simulink model "Buck_DCM_s"  (R2020a)
settings: Solver=FixedStepAuto  StartTime=0.0  StopTime=1  FixedStep=T  RelTol=1e-3
undefined symbols (not defined in the file): C, Idm, Iumax, J, Ki_I, Ki_IL, Ki_W, Kp_I, Kp_IL, Kp_Uc, Kp_W, Kphi, L, Lu, rL, Ru, Ubat
libraries: fl_lib x7, simulink x6, nesl_utility x3, powerlib_meascontrol x2
settings Model: SILPILModeSetting=veronly  ExtModeTrigDuration=2  Creator=Nguyễn Thanh Tùng  LastModifiedBy=Nguyen Tung
settings OptimizationCC: DefaultParameterBehavior=Inlined  EnhancedBackFolding=on  PassReuseOutputArgsAs=Individual arguments  ZeroExternalMemoryAtStartup=off  ZeroInternalMemoryAtStartup=off  MaxStackSize=64  OptimizeBlockOrder=speed  DifferentSizesBufferReuse=on  OptimizationCustomize=off  EfficientTunableParamExpr=on
settings DebuggingCC: ParameterTunabilityLossMsg=error
settings SFSimCC: MATLABDynamicMemAlloc=off  CustomCodeUndefinedFunction=UseInterfaceOnly
settings RTWCC: SystemTargetFile=ert.tlc  TemplateMakefile=ert_default_tmf  Toolchain=Arduino ARM  BuildConfiguration=Faster Runs
settings CodeAppCC: ForceParamTrailComments=on  IgnoreCustomStorageClasses=off  OperatorAnnotations=on  SimulinkDataObjDesc=on  SFDataObjDesc=on  InsertBlockDesc=on
settings ERTTargetCC: SupportContinuousTime=on  ExtModeStaticAllocSize=24576  ERTCustomFileTemplate=example_file_process.tlc

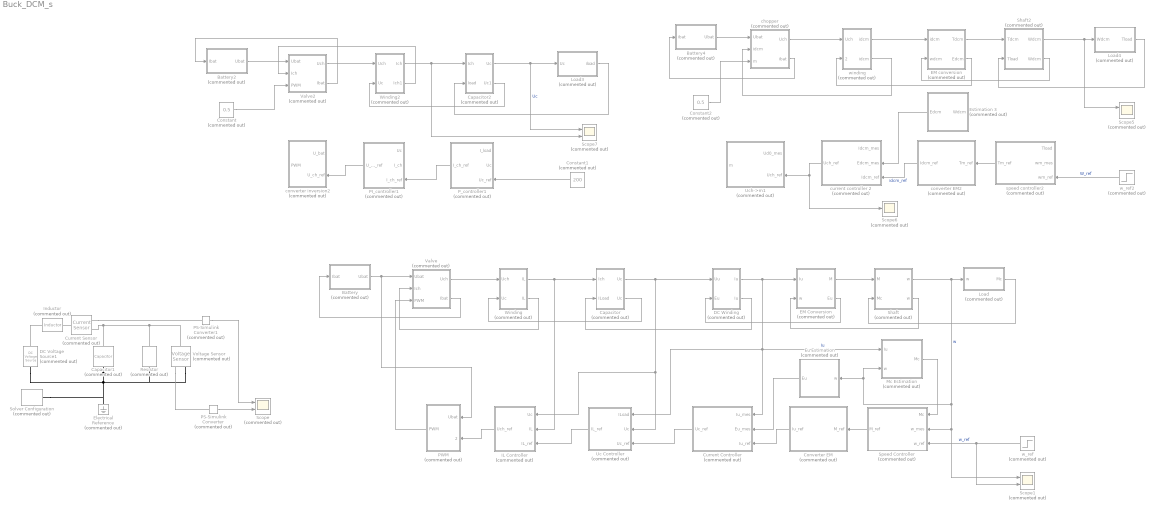
== system Buck_DCM_s ==
  Battery : Subsystem  Commented=on  AncestorBlock=simulink/REM/SE
      mask Display:
      | plot(0,0,100,100, 1.2*[50,57.68,60.77,63.08,64.97,66.58,68,69.26,70.4, 	71.42,72.36,78.28,80,78.28,72.36,71.42,70.4, 	69.26,68,66.58,64.97,63.08,60.77,57.68,50,42.32, 	39.23,36.92,35.03,33.42,32,30.74,29.6,28.58, 	27.64,21.72,20,21.72,27.64,28.58,29.6,30.74,32, 	33.42,35.03,36.92,39.23,42.32,50]-10, 1.2*[20,21,22,23,24,25,26,27,28,29,30,40,50,60,70,71,72, 	73,74,75,76,77,78,79,80,79,78,77,76,75,74,73,72, 	71,70,60,50,40,30,29,28,27,26,25,24,23,22,21,20]-10)
      | disp('ES')
  Battery2 : Subsystem  Commented=on  AncestorBlock=simulink/REM/SE
      mask Display:
      | plot(0,0,100,100, 1.2*[50,57.68,60.77,63.08,64.97,66.58,68,69.26,70.4, 	71.42,72.36,78.28,80,78.28,72.36,71.42,70.4, 	69.26,68,66.58,64.97,63.08,60.77,57.68,50,42.32, 	39.23,36.92,35.03,33.42,32,30.74,29.6,28.58, 	27.64,21.72,20,21.72,27.64,28.58,29.6,30.74,32, 	33.42,35.03,36.92,39.23,42.32,50]-10, 1.2*[20,21,22,23,24,25,26,27,28,29,30,40,50,60,70,71,72, 	73,74,75,76,77,78,79,80,79,78,77,76,75,74,73,72, 	71,70,60,50,40,30,29,28,27,26,25,24,23,22,21,20]-10)
      | disp('ES')
  Battery4 : Subsystem  Commented=on  AncestorBlock=simulink/REM/SE
      mask Display:
      | plot(0,0,100,100, 1.2*[50,57.68,60.77,63.08,64.97,66.58,68,69.26,70.4, 	71.42,72.36,78.28,80,78.28,72.36,71.42,70.4, 	69.26,68,66.58,64.97,63.08,60.77,57.68,50,42.32, 	39.23,36.92,35.03,33.42,32,30.74,29.6,28.58, 	27.64,21.72,20,21.72,27.64,28.58,29.6,30.74,32, 	33.42,35.03,36.92,39.23,42.32,50]-10, 1.2*[20,21,22,23,24,25,26,27,28,29,30,40,50,60,70,71,72, 	73,74,75,76,77,78,79,80,79,78,77,76,75,74,73,72, 	71,70,60,50,40,30,29,28,27,26,25,24,23,22,21,20]-10)
      | disp('ES')
  Capacitor : Subsystem  Commented=on  AncestorBlock=simulink/REM/EA  mask(CM){}
      mask Display: plot(0,0,100,100,[10,10,90,90,10],[90,10,10,90,90], [10,90],[10,90])
  Capacitor1 : fl_lib/Electrical/Electrical Elements/Capacitor  Commented=on  c=C F  r=0 Ohm  g=0 1/Ohm  i_specify=off  i_priority=None  i=0 A  i_nominal_specify=off  i_nominal_unit=A  i_nominal_value=1  v_specify=off  v_priority=None  v=0 V  v_nominal_specify=off  v_nominal_unit=V  v_nominal_value=1  vc_specify=off  vc_priority=High  vc=0 V  vc_nominal_specify=off  vc_nominal_unit=V  vc_nominal_value=1
  Capacitor2 : Subsystem  Commented=on  AncestorBlock=simulink/REM/EA  mask(CM){}
      mask Display: plot(0,0,100,100,[10,10,90,90,10],[90,10,10,90,90], [10,90],[10,90])
  Constant : Constant  Commented=on  Value=0.5
  Constant1 : Constant  Commented=on  Value=200
  Constant2 : Constant  Commented=on  Value=0.5
  Converter EM : Subsystem  Commented=on  AncestorBlock=simulink/SMC/Inversion EC avec mesure
      mask Display: plot(0,0,100,100,[10,30,90,70,10],[90,10,10,90,90])
  Current Controller : Subsystem  Commented=on  AncestorBlock=simulink/SMC/Asservissement Correcteur IP
      mask Display: plot(0,0,100,100, [10,30,90,70,10,90],[90,10,10,90,90,10])
  Current Sensor : fl_lib/Electrical/Electrical Sensors/Current Sensor  Commented=on
  DC Voltage Source1 : fl_lib/Electrical/Electrical Sources/DC Voltage Source  Commented=on  v0=100 V
  DC Winding : Subsystem  Commented=on  AncestorBlock=simulink/REM/EA  mask(CM){}
      mask Display: plot(0,0,100,100,[10,10,90,90,10],[90,10,10,90,90], [10,90],[10,90])
  EM Conversion : Subsystem  Commented=on  AncestorBlock=simulink/REM/EC EM
      mask Display: plot(0,0,100,100, 1.4*[50,57.68,60.77,63.08,64.97,66.58,68,69.26,70.4, 	71.42,72.36,78.28,80,78.28,72.36,71.42,70.4, 	69.26,68,66.58,64.97,63.08,60.77,57.68,50,42.32, 	39.23,36.92,35.03,33.42,32,30.74,29.6,28.58, 	27.64,21.72,20,21.72,27.64,28.58,29.6,30.74,32, 	33.42,35.03,36.92,39.23,42.32,50]-20, 1.4*[20,21,22,23,24,25,26,27,28,29,30,40,50,60,70,71,72, 	73,74,75,76,77,78,79,80,79,78,77,76,75,74,73,72, 	71,70,60,50,40,30,29,28,27,26,25,24,23,22,21,20]-20)
  EM conversion : Subsystem  Commented=on  AncestorBlock=simulink/REM/EC EM
      mask Display: plot(0,0,100,100, 1.4*[50,57.68,60.77,63.08,64.97,66.58,68,69.26,70.4, 	71.42,72.36,78.28,80,78.28,72.36,71.42,70.4, 	69.26,68,66.58,64.97,63.08,60.77,57.68,50,42.32, 	39.23,36.92,35.03,33.42,32,30.74,29.6,28.58, 	27.64,21.72,20,21.72,27.64,28.58,29.6,30.74,32, 	33.42,35.03,36.92,39.23,42.32,50]-20, 1.4*[20,21,22,23,24,25,26,27,28,29,30,40,50,60,70,71,72, 	73,74,75,76,77,78,79,80,79,78,77,76,75,74,73,72, 	71,70,60,50,40,30,29,28,27,26,25,24,23,22,21,20]-20)
  Electrical Reference : fl_lib/Electrical/Electrical Elements/Electrical Reference  Commented=on
  Estimation 3 : Subsystem  Commented=on  AncestorBlock=simulink/REM/EC EM
      mask Display: plot(0,0,100,100, 1.4*[50,57.68,60.77,63.08,64.97,66.58,68,69.26,70.4, 	71.42,72.36,78.28,80,78.28,72.36,71.42,70.4, 	69.26,68,66.58,64.97,63.08,60.77,57.68,50,42.32, 	39.23,36.92,35.03,33.42,32,30.74,29.6,28.58, 	27.64,21.72,20,21.72,27.64,28.58,29.6,30.74,32, 	33.42,35.03,36.92,39.23,42.32,50]-20, 1.4*[20,21,22,23,24,25,26,27,28,29,30,40,50,60,70,71,72, 	73,74,75,76,77,78,79,80,79,78,77,76,75,74,73,72, 	71,70,60,50,40,30,29,28,27,26,25,24,23,22,21,20]-20)
  Eu Estimation : Subsystem  Commented=on  AncestorBlock=simulink/REM/EC EM
      mask Display: plot(0,0,100,100, 1.4*[50,57.68,60.77,63.08,64.97,66.58,68,69.26,70.4, 	71.42,72.36,78.28,80,78.28,72.36,71.42,70.4, 	69.26,68,66.58,64.97,63.08,60.77,57.68,50,42.32, 	39.23,36.92,35.03,33.42,32,30.74,29.6,28.58, 	27.64,21.72,20,21.72,27.64,28.58,29.6,30.74,32, 	33.42,35.03,36.92,39.23,42.32,50]-20, 1.4*[20,21,22,23,24,25,26,27,28,29,30,40,50,60,70,71,72, 	73,74,75,76,77,78,79,80,79,78,77,76,75,74,73,72, 	71,70,60,50,40,30,29,28,27,26,25,24,23,22,21,20]-20)
  IL Controller : Subsystem  Commented=on  AncestorBlock=simulink/SMC/Asservissement Correcteur IP
      mask Display: plot(0,0,100,100, [10,30,90,70,10,90],[90,10,10,90,90,10])
  Inductor : fl_lib/Electrical/Electrical Elements/Inductor  Commented=on  l=L H  r=rL Ohm  g=0 1/Ohm  i_specify=off  i_priority=None  i=0 A  i_nominal_specify=off  i_nominal_unit=A  i_nominal_value=1  v_specify=off  v_priority=None  v=0 V  v_nominal_specify=off  v_nominal_unit=V  v_nominal_value=1  i_L_specify=off  i_L_priority=High  i_L=0 A  i_L_nominal_specify=off  i_L_nominal_unit=A  i_L_nominal_value=1
  Load : Subsystem  Commented=on  AncestorBlock=simulink/REM/SE
      mask Display:
      | plot(0,0,100,100, 1.2*[50,57.68,60.77,63.08,64.97,66.58,68,69.26,70.4, 	71.42,72.36,78.28,80,78.28,72.36,71.42,70.4, 	69.26,68,66.58,64.97,63.08,60.77,57.68,50,42.32, 	39.23,36.92,35.03,33.42,32,30.74,29.6,28.58, 	27.64,21.72,20,21.72,27.64,28.58,29.6,30.74,32, 	33.42,35.03,36.92,39.23,42.32,50]-10, 1.2*[20,21,22,23,24,25,26,27,28,29,30,40,50,60,70,71,72, 	73,74,75,76,77,78,79,80,79,78,77,76,75,74,73,72, 	71,70,60,50,40,30,29,28,27,26,25,24,23,22,21,20]-10)
      | disp('MS')
  Load3 : Subsystem  Commented=on  AncestorBlock=simulink/REM/SE
      mask Display:
      | plot(0,0,100,100, 1.2*[50,57.68,60.77,63.08,64.97,66.58,68,69.26,70.4, 	71.42,72.36,78.28,80,78.28,72.36,71.42,70.4, 	69.26,68,66.58,64.97,63.08,60.77,57.68,50,42.32, 	39.23,36.92,35.03,33.42,32,30.74,29.6,28.58, 	27.64,21.72,20,21.72,27.64,28.58,29.6,30.74,32, 	33.42,35.03,36.92,39.23,42.32,50]-10, 1.2*[20,21,22,23,24,25,26,27,28,29,30,40,50,60,70,71,72, 	73,74,75,76,77,78,79,80,79,78,77,76,75,74,73,72, 	71,70,60,50,40,30,29,28,27,26,25,24,23,22,21,20]-10)
      | disp('ES')
  Load4 : Subsystem  Commented=on  AncestorBlock=simulink/REM/SE
      mask Display:
      | plot(0,0,100,100, 1.2*[50,57.68,60.77,63.08,64.97,66.58,68,69.26,70.4, 	71.42,72.36,78.28,80,78.28,72.36,71.42,70.4, 	69.26,68,66.58,64.97,63.08,60.77,57.68,50,42.32, 	39.23,36.92,35.03,33.42,32,30.74,29.6,28.58, 	27.64,21.72,20,21.72,27.64,28.58,29.6,30.74,32, 	33.42,35.03,36.92,39.23,42.32,50]-10, 1.2*[20,21,22,23,24,25,26,27,28,29,30,40,50,60,70,71,72, 	73,74,75,76,77,78,79,80,79,78,77,76,75,74,73,72, 	71,70,60,50,40,30,29,28,27,26,25,24,23,22,21,20]-10)
      | disp('MS')
  Mc Estimation : Subsystem  Commented=on  AncestorBlock=simulink/REM/EC EM
      mask Display: plot(0,0,100,100, 1.4*[50,57.68,60.77,63.08,64.97,66.58,68,69.26,70.4, 	71.42,72.36,78.28,80,78.28,72.36,71.42,70.4, 	69.26,68,66.58,64.97,63.08,60.77,57.68,50,42.32, 	39.23,36.92,35.03,33.42,32,30.74,29.6,28.58, 	27.64,21.72,20,21.72,27.64,28.58,29.6,30.74,32, 	33.42,35.03,36.92,39.23,42.32,50]-20, 1.4*[20,21,22,23,24,25,26,27,28,29,30,40,50,60,70,71,72, 	73,74,75,76,77,78,79,80,79,78,77,76,75,74,73,72, 	71,70,60,50,40,30,29,28,27,26,25,24,23,22,21,20]-20)
  PI_controller1 : Subsystem  Commented=on  AncestorBlock=simulink/SMC/Asservissement Correcteur IP
      mask Display: plot(0,0,100,100, [10,30,90,70,10,90],[90,10,10,90,90,10])
  PS-Simulink Converter : nesl_utility/PS-Simulink Converter  Commented=on  PhysicalDomain=network_engine_domain  SubClassName=ps_output  LeftPortType=input  RightPortType=output  PseudoPeriodic=off  Frequencies=[]  Unit=inherit  AffineConversion=off
  PS-Simulink Converter1 : nesl_utility/PS-Simulink Converter  Commented=on  PhysicalDomain=network_engine_domain  SubClassName=ps_output  LeftPortType=input  RightPortType=output  PseudoPeriodic=off  Frequencies=[]  Unit=inherit  AffineConversion=off
  PWM : Subsystem  Commented=on  AncestorBlock=simulink/SMC/Inversion EC avec mesure
      mask Display: plot(0,0,100,100,[10,30,90,70,10],[90,10,10,90,90])
  P_controller1 : Subsystem  Commented=on  AncestorBlock=simulink/SMC/Asservissement Correcteur IP
      mask Display: plot(0,0,100,100, [10,30,90,70,10,90],[90,10,10,90,90,10])
  Resistor : fl_lib/Electrical/Electrical Elements/Resistor  Commented=on  R=10 Ohm  i_specify=off  i_priority=None  i=0 A  i_nominal_specify=off  i_nominal_unit=A  i_nominal_value=1  v_specify=off  v_priority=None  v=0 V  v_nominal_specify=off  v_nominal_unit=V  v_nominal_value=1
  Scope{,1,5,7} (4 alike) : Scope  Commented=on  NumInputPorts=2
  Scope6 : Scope  Commented=on
  Shaft : Subsystem  Commented=on  AncestorBlock=simulink/REM/EA  mask(CM){}
      mask Display: plot(0,0,100,100,[10,10,90,90,10],[90,10,10,90,90], [10,90],[10,90])
  Shaft2 : Subsystem  Commented=on  AncestorBlock=simulink/REM/EA  mask(CM){}
      mask Display: plot(0,0,100,100,[10,10,90,90,10],[90,10,10,90,90], [10,90],[10,90])
  Solver Configuration : nesl_utility/Solver Configuration  Commented=on  PhysicalDomain=network_engine_domain  SubClassName=solver  LeftPortType=input  RightPortType=generic  Tones=[]  Harmonics=[]  SimulateNoise=off  Profile=off  UseLocalSampling=off  EnableSwitchedLinearOptims=on  FrequencyDomain=off  UseCCode=off  RelTol=0.001  AbsTol=1e-06  MinStep=1e-09  ToWorkspace=off  RevertToSquareIcSolve=off  NumHomotopyIterations=100  PhasorMode=off  PhasorModeNumHarmonics=1  DoDC=off  ResidualTolerance=1e-09  UseLocalSolver=off  LocalSolverChoice=NE_BACKWARD_EULER_ADVANCER  LocalSolverSampleTime=0.001  DoFixedCost=off  MaxNonlinIter=3  MaxModeIter=2  LinearAlgebra=auto  EquationFormulation=NE_TIME_EF  DelaysMemoryBudget=1024  AutomaticFiltering=on  FilteringTimeConstant=0.001  PartitionStorageMethod=AS_NEEDED  PartitionMemoryBudget=1024  PartitionMethod=ROBUST
  Speed Controller : Subsystem  Commented=on  AncestorBlock=simulink/SMC/Asservissement Correcteur IP
      mask Display: plot(0,0,100,100, [10,30,90,70,10,90],[90,10,10,90,90,10])
  Uc Controller : Subsystem  Commented=on  AncestorBlock=simulink/SMC/Asservissement Correcteur IP
      mask Display: plot(0,0,100,100, [10,30,90,70,10,90],[90,10,10,90,90,10])
  Uch->m1 : Subsystem  Commented=on  AncestorBlock=simulink/SMC/Inversion EC avec mesure
      mask Display: plot(0,0,100,100,[10,30,90,70,10],[90,10,10,90,90])
  Valve : Subsystem  Commented=on  AncestorBlock=simulink/REM/EC Elec  mask(Hacheur){}
      mask Display: plot(0,0,100,100,[10,10,90,90,10],[90,10,10,90,90])
  Valve2 : Subsystem  Commented=on  AncestorBlock=simulink/REM/EC Elec  mask(Hacheur){}
      mask Display: plot(0,0,100,100,[10,10,90,90,10],[90,10,10,90,90])
  Voltage Sensor : fl_lib/Electrical/Electrical Sensors/Voltage Sensor  Commented=on
  Winding : Subsystem  Commented=on  AncestorBlock=simulink/REM/EA  mask(CM){}
      mask Display: plot(0,0,100,100,[10,10,90,90,10],[90,10,10,90,90], [10,90],[10,90])
  Winding2 : Subsystem  Commented=on  AncestorBlock=simulink/REM/EA  mask(CM){}
      mask Display: plot(0,0,100,100,[10,10,90,90,10],[90,10,10,90,90], [10,90],[10,90])
  chopper : Subsystem  Commented=on  AncestorBlock=simulink/REM/EC Elec  mask(Hacheur){}
      mask Display: plot(0,0,100,100,[10,10,90,90,10],[90,10,10,90,90])
  converter EM2 : Subsystem  Commented=on  AncestorBlock=simulink/SMC/Inversion EC avec mesure
      mask Display: plot(0,0,100,100,[10,30,90,70,10],[90,10,10,90,90])
  converter inversion2 : Subsystem  Commented=on  AncestorBlock=simulink/SMC/Inversion EC avec mesure
      mask Display: plot(0,0,100,100,[10,30,90,70,10],[90,10,10,90,90])
  current controller 2 : Subsystem  Commented=on  AncestorBlock=simulink/SMC/Asservissement Correcteur IP
      mask Display: plot(0,0,100,100, [10,30,90,70,10,90],[90,10,10,90,90,10])
  speed controller2 : Subsystem  Commented=on  AncestorBlock=simulink/SMC/Asservissement Correcteur IP
      mask Display: plot(0,0,100,100, [10,30,90,70,10,90],[90,10,10,90,90,10])
  w_ref : Step  Commented=on  Time=0  After=100  SampleTime=0
  w_ref2 : Step  Commented=on  Time=0.01  After=50  SampleTime=0
  winding : Subsystem  Commented=on  AncestorBlock=simulink/REM/EA  mask(CM){}
      mask Display: plot(0,0,100,100,[10,10,90,90,10],[90,10,10,90,90], [10,90],[10,90])
  wires:
  Speed Controller/1(M_ref) -> Converter EM/1(M_ref)
  Capacitor/1(Uc) -> DC Winding/1(Uu), IL Controller/1(Uc), Uc Controller/2(Uc)
  EM Conversion/1(M) -> Shaft/1(M)
  DC Winding/1("Iu ") -> Uc Controller/1(ILoad), Mc Estimation/1(Iu), Current Controller/1(Iu_mes), EM Conversion/1(Iu)  "Iu"
  Eu Estimation/1(Eu) -> Current Controller/2(Eu_mes)
  DC Winding/2(Iu) -> Capacitor/2(ILoad)
  Converter EM/1(Iu_ref) -> Current Controller/3(Iu_ref)
  Capacitor/2("Uc ") -> Winding/2(Uc)
  w_ref/1 -> Speed Controller/3(w_ref), Scope1/2  "w_ref"
  Winding/1(IL) -> Capacitor/1(Ich), IL Controller/2(IL)
  Load/1(Mc) -> Shaft/2(Mc)
  EM Conversion/2(Eu) -> DC Winding/2(Eu)
  PWM/1(PWM) -> Valve/3(PWM)
  Valve/2(Ibat) -> Battery/1(Ibat)
  Battery/1(Ubat) -> PWM/1(Ubat), Valve/1(Ubat)
  Shaft/2("w ") -> EM Conversion/2(w)
  Shaft/1(w) -> Scope1/1, Speed Controller/2(w_mes), Mc Estimation/2(w), Eu Estimation/1(w), Load/1(w)  "w"
  Uc Controller/1(IL_ref) -> IL Controller/3(IL_ref)
  IL Controller/1(Uch_ref) -> PWM/2(Uch_ref)
  chopper/1(Uch) -> winding/1(Uch)
  EM conversion/2(Edcm) -> winding/2(Edcm)
  winding/2(idcm) -> chopper/2(idcm)
  Load4/1(Tload) -> Shaft2/2(Tload)
  chopper/2(ibat) -> Battery4/1(ibat)
  Battery2/1(Ubat) -> Valve2/1(Ubat)
  P_controller1/1(I_ch_ref) -> PI_controller1/3("I_ch_ref ")
  Load3/1(iload) -> Capacitor2/2(Ioad)
  Valve2/1(Uch) -> Winding2/1(Uch)
  Battery4/1(Ubat) -> chopper/1("Ubat ")
  Capacitor2/2(Uc1) -> Winding2/2(Uc)
  w_ref2/1 -> speed controller2/3(wm_ref)  "W_ref"
  winding/1("idcm ") -> EM conversion/1(idcm)
  Winding2/2(Ich1) -> Valve2/2(Ich)
  Shaft2/2("Wdcm ") -> EM conversion/2(wdcm)
  EM conversion/1(Tdcm) -> Shaft2/1(Tdcm)
  PI_controller1/1(U_ch_ref) -> converter inversion2/2(U_ch_ref)
  Shaft2/1(Wdcm) -> Scope5/1, Load4/1(Wdcm)
  Winding2/1(Ich) -> Scope7/2, Capacitor2/1(Ich)
  Capacitor2/1(Uc) -> Scope7/1, Load3/1(Uc)  "Uc"
  speed controller2/1(Tm_ref) -> converter EM2/1(Tm_ref)
  current controller 2/1(Uch_ref) -> Uch->m1/2(Uch_ref), Scope6/1
  Estimation 3/1(Edcm) -> current controller 2/2(Edcm_mes)
  Constant1/1 -> P_controller1/3(Uc_ref)
  converter EM2/1(Idcm_ref) -> current controller 2/3(Idcm_ref)  "idcm_ref"
  Valve2/2(Ibat) -> Battery2/1(Ibat)
  Valve/1(Uch) -> Winding/1(Uch)
  Current Controller/1(Uc_ref) -> Uc Controller/3(Uc_ref)
  Winding/2("IL ") -> Valve/2(Ich)
  Mc Estimation/1(Mc) -> Speed Controller/1(Mc)
  Constant/1 -> Valve2/3(PWM)
  Constant2/1 -> chopper/3(m)
  PS-Simulink Converter1/1 -> Scope/1
  PS-Simulink Converter/1 -> Scope/2
  connections:
  DC Voltage Source1/LConn1 -- Inductor/LConn1
  Resistor/LConn1 -- Voltage Sensor/LConn1 -- Current Sensor/RConn2 -- Capacitor1/LConn1
  Capacitor1/RConn1 -- DC Voltage Source1/RConn1 -- Solver Configuration/RConn1 -- Electrical Reference/LConn1 -- Voltage Sensor/RConn2 -- Resistor/RConn1
  Voltage Sensor/RConn1 -- PS-Simulink Converter/LConn1
  Current Sensor/LConn1 -- Inductor/RConn1
  Current Sensor/RConn1 -- PS-Simulink Converter1/LConn1

== system Buck_DCM_s/Battery ==
  Ibat : Inport
  Constant : Constant  Value=Ubat
  Terminator : Terminator
  Ubat : Outport  InitialOutput=0  VectorParamsAs1DForOutWhenUnconnected=off
  wires:
  Constant/1 -> Ubat/1
  Ibat/1 -> Terminator/1

== system Buck_DCM_s/Battery2 ==
  Ibat : Inport
  Constant : Constant  Value=Ubat
  Terminator : Terminator
  Ubat : Outport  InitialOutput=0  VectorParamsAs1DForOutWhenUnconnected=off
  wires:
  Constant/1 -> Ubat/1
  Ibat/1 -> Terminator/1

== system Buck_DCM_s/Battery4 ==
  ibat : Inport
  Terminator : Terminator
  U_bat : Constant  Value=Ubat
  Ubat : Outport  InitialOutput=0  VectorParamsAs1DForOutWhenUnconnected=off
  wires:
  ibat/1 -> Terminator/1
  U_bat/1 -> Ubat/1

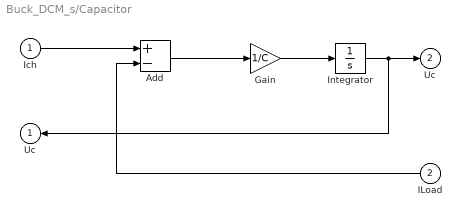
== system Buck_DCM_s/Capacitor ==
  Ich : Inport
  ILoad : Inport  Port=2
  Add : Sum  Inputs=+-
  Gain : Gain  Gain=1/C
  Integrator : Integrator
  Uc : Outport  InitialOutput=0  VectorParamsAs1DForOutWhenUnconnected=off
  "Uc " : Outport  Port=2  InitialOutput=0  VectorParamsAs1DForOutWhenUnconnected=off
  wires:
  Ich/1 -> Add/1
  Add/1 -> Gain/1
  Gain/1 -> Integrator/1
  Integrator/1 -> "Uc "/1, Uc/1
  ILoad/1 -> Add/2

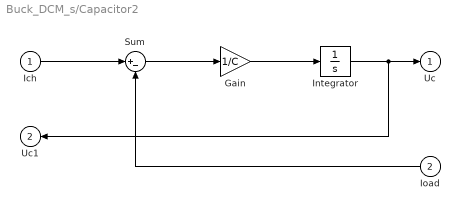
== system Buck_DCM_s/Capacitor2 ==
  Ich : Inport
  Ioad : Inport  Port=2
  Gain : Gain  Gain=1/C
  Integrator : Integrator
  Sum : Sum  Inputs=|+-
  Uc : Outport  InitialOutput=0  VectorParamsAs1DForOutWhenUnconnected=off
  Uc1 : Outport  Port=2  InitialOutput=0  VectorParamsAs1DForOutWhenUnconnected=off
  wires:
  Ich/1 -> Sum/1
  Sum/1 -> Gain/1
  Gain/1 -> Integrator/1
  Integrator/1 -> Uc1/1, Uc/1
  Ioad/1 -> Sum/2

== system Buck_DCM_s/Converter EM ==
  M_ref : Inport
  Gain : Gain  Gain=1/Kphi
  Saturation : Saturate  UpperLimit=Iumax  LowerLimit=0
  Iu_ref : Outport  InitialOutput=0  VectorParamsAs1DForOutWhenUnconnected=off
  wires:
  M_ref/1 -> Gain/1
  Gain/1 -> Saturation/1
  Saturation/1 -> Iu_ref/1

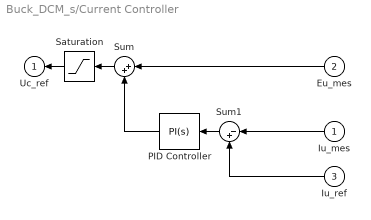
== system Buck_DCM_s/Current Controller ==
  Iu_mes : Inport
  Eu_mes : Inport  Port=2
  Iu_ref : Inport  Port=3
  PID Controller : simulink/Continuous/PID Controller  Controller=PI  Form=Parallel  TimeDomain=Continuous-time  UseExternalTs=off  SampleTime=-1  IntegratorMethod=Forward Euler  FilterMethod=Forward Euler  ControllerParametersSource=internal  P=Kp_I  I=Ki_I  D=0  UseFilter=on  N=100  TunerSelectOption=Transfer Function Based (PID Tuner App)  InitialConditionSource=internal  InitialConditionForIntegrator=0  InitialConditionForFilter=0  DifferentiatorICPrevScaledInput=0  ExternalReset=none  IgnoreLimit=on  TrackingMode=off  Kt=1  LimitOutput=off  UpperSaturationLimit=inf  LowerSaturationLimit=-inf  LinearizeAsGain=on  AntiWindupMode=none  Kb=1  POutMin=[]  POutMax=[]  IOutMin=[]  IOutMax=[]  DOutMin=[]  DOutMax=[]  NOutMin=[]  NOutMax=[]  SumOutMin=[]  SumOutMax=[]  SaturationOutMin=[]  SaturationOutMax=[]  PParamMin=[]  PParamMax=[]  IParamMin=[]  IParamMax=[]  DParamMin=[]  DParamMax=[]  NParamMin=[]  NParamMax=[]  KbParamMin=[]  KbParamMax=[]  KtParamMin=[]  KtParamMax=[]  KbOutMin=[]  KbOutMax=[]  KtOutMin=[]  KtOutMax=[]  IntegratorOutMin=[]  IntegratorOutMax=[]  FilterOutMin=[]  FilterOutMax=[]  SumI1OutMin=[]  SumI1OutMax=[]  SumI2OutMin=[]  SumI2OutMax=[]  SumI3OutMin=[]  SumI3OutMax=[]  SumI4OutMin=[]  SumI4OutMax=[]  SumDOutMin=[]  SumDOutMax=[]  DifferentiatorOutMin=[]  DifferentiatorOutMax=[]  FilterDiffOutCoefMin=[]  FilterDiffOutCoefMax=[]  ReciprocalOutMin=[]  ReciprocalOutMax=[]  SumDenOutMin=[]  SumDenOutMax=[]  SumNumOutMin=[]  SumNumOutMax=[]  DivideOutMin=[]  DivideOutMax=[]  UdiffTsProdOutMin=[]  UdiffTsProdOutMax=[]  NTsProdOutMin=[]  NTsProdOutMax=[]  UintegralTsProdOutMin=[]  UintegralTsProdOutMax=[]  UngainTsProdOutMin=[]  UngainTsProdOutMax=[]  IntegratorContinuousStateAttributes=''  IntegratorStateMustResolveToSignalObject=off  IntegratorRTWStateStorageClass=Auto  FilterContinuousStateAttributes=''  FilterStateMustResolveToSignalObject=off  FilterRTWStateStorageClass=Auto  ParallelPVariant=InternalParameters  IdealPVariant=Disabled  IVariant=InternalParameters  DVariant=Disabled  IntegratorVariant=Continuous  SatVariant=Disabled  AWVariant=Passthrough  PCopyVariant=Disabled  TRVariant=Disabled  FdbkBlocksVariant=Forward  IdealPFdbkVariant=Disabled  SatFdbkVariant=Disabled  DerivativeFilterVariant=Disabled  NVariant=Disabled  NCopyVariant=Disabled_SignalSpec  FilterICVariant=Disabled  IntegratorICVariant=InternalICs  ExternalResetVariant=Disabled  TRSumVariant=Passthrough  SumFdbkVariant=Disabled  SumVariant=Sum_PI  TsampFilterVariant=InternalTs  TsampNgainVariant=Passthrough  TsampIntegralVariant=Passthrough
  Saturation : Saturate  UpperLimit=400  LowerLimit=0
  Sum : Sum  Inputs=|++
  Sum1 : Sum  Inputs=|-+
  Uc_ref : Outport  InitialOutput=0  VectorParamsAs1DForOutWhenUnconnected=off
  wires:
  Eu_mes/1 -> Sum/1
  Sum/1 -> Saturation/1
  Iu_mes/1 -> Sum1/1
  Sum1/1 -> PID Controller/1
  PID Controller/1 -> Sum/2
  Iu_ref/1 -> Sum1/2
  Saturation/1 -> Uc_ref/1

== system Buck_DCM_s/DC Winding ==
  Uu : Inport
  Eu : Inport  Port=2
  1/(Ls+R) : TransferFcn  Denominator=[Lu Ru]
  Sum : Sum  Inputs=|+-
  "Iu " : Outport  InitialOutput=0  VectorParamsAs1DForOutWhenUnconnected=off
  Iu : Outport  Port=2  InitialOutput=0  VectorParamsAs1DForOutWhenUnconnected=off
  wires:
  Uu/1 -> Sum/1
  Eu/1 -> Sum/2
  Sum/1 -> 1/(Ls+R)/1
  1/(Ls+R)/1 -> Iu/1, "Iu "/1

== system Buck_DCM_s/EM Conversion ==
  Iu : Inport
  w : Inport  Port=2
  Gain : Gain  Gain=Kphi
  Gain1 : Gain  Gain=Kphi
  M : Outport  InitialOutput=0  VectorParamsAs1DForOutWhenUnconnected=off
  Eu : Outport  Port=2  InitialOutput=0  VectorParamsAs1DForOutWhenUnconnected=off
  wires:
  Iu/1 -> Gain/1
  Gain/1 -> M/1
  w/1 -> Gain1/1
  Gain1/1 -> Eu/1

== system Buck_DCM_s/EM conversion ==
  idcm : Inport
  wdcm : Inport  Port=2
  Gain : Gain  Gain=Kphi
  Gain1 : Gain  Gain=Kphi
  Tdcm : Outport  InitialOutput=0  VectorParamsAs1DForOutWhenUnconnected=off
  Edcm : Outport  Port=2  InitialOutput=0  VectorParamsAs1DForOutWhenUnconnected=off
  wires:
  idcm/1 -> Gain/1
  Gain/1 -> Tdcm/1
  wdcm/1 -> Gain1/1
  Gain1/1 -> Edcm/1

== system Buck_DCM_s/Estimation 3 ==
  Wdcm : Inport
  Gain1 : Gain  Gain=Kphi
  Edcm : Outport  InitialOutput=0  VectorParamsAs1DForOutWhenUnconnected=off
  wires:
  Wdcm/1 -> Gain1/1
  Gain1/1 -> Edcm/1

== system Buck_DCM_s/Eu Estimation ==
  w : Inport
  Gain1 : Gain  Gain=Kphi
  Eu : Outport  InitialOutput=0  VectorParamsAs1DForOutWhenUnconnected=off
  wires:
  w/1 -> Gain1/1
  Gain1/1 -> Eu/1

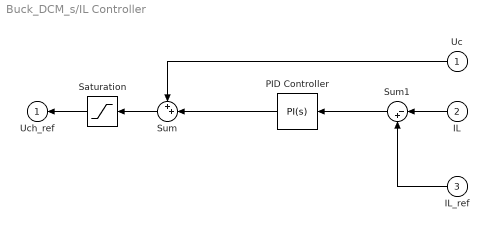
== system Buck_DCM_s/IL Controller ==
  Uc : Inport
  IL : Inport  Port=2
  IL_ref : Inport  Port=3
  PID Controller : simulink/Continuous/PID Controller  Controller=PI  Form=Parallel  TimeDomain=Continuous-time  UseExternalTs=off  SampleTime=-1  IntegratorMethod=Forward Euler  FilterMethod=Forward Euler  ControllerParametersSource=internal  P=Kp_IL  I=Ki_IL  D=0  UseFilter=on  N=100  TunerSelectOption=Transfer Function Based (PID Tuner App)  InitialConditionSource=internal  InitialConditionForIntegrator=0  InitialConditionForFilter=0  DifferentiatorICPrevScaledInput=0  ExternalReset=none  TrackingMode=off  Kt=1  LimitOutput=off  UpperSaturationLimit=inf  LowerSaturationLimit=-inf  LinearizeAsGain=on  AntiWindupMode=none  Kb=1  POutMin=[]  POutMax=[]  IOutMin=[]  IOutMax=[]  DOutMin=[]  DOutMax=[]  NOutMin=[]  NOutMax=[]  SumOutMin=[]  SumOutMax=[]  SaturationOutMin=[]  SaturationOutMax=[]  PParamMin=[]  PParamMax=[]  IParamMin=[]  IParamMax=[]  DParamMin=[]  DParamMax=[]  NParamMin=[]  NParamMax=[]  KbParamMin=[]  KbParamMax=[]  KtParamMin=[]  KtParamMax=[]  KbOutMin=[]  KbOutMax=[]  KtOutMin=[]  KtOutMax=[]  IntegratorOutMin=[]  IntegratorOutMax=[]  FilterOutMin=[]  FilterOutMax=[]  SumI1OutMin=[]  SumI1OutMax=[]  SumI2OutMin=[]  SumI2OutMax=[]  SumI3OutMin=[]  SumI3OutMax=[]  SumI4OutMin=[]  SumI4OutMax=[]  SumDOutMin=[]  SumDOutMax=[]  DifferentiatorOutMin=[]  DifferentiatorOutMax=[]  FilterDiffOutCoefMin=[]  FilterDiffOutCoefMax=[]  ReciprocalOutMin=[]  ReciprocalOutMax=[]  SumDenOutMin=[]  SumDenOutMax=[]  SumNumOutMin=[]  SumNumOutMax=[]  DivideOutMin=[]  DivideOutMax=[]  UdiffTsProdOutMin=[]  UdiffTsProdOutMax=[]  NTsProdOutMin=[]  NTsProdOutMax=[]  UintegralTsProdOutMin=[]  UintegralTsProdOutMax=[]  UngainTsProdOutMin=[]  UngainTsProdOutMax=[]  IntegratorContinuousStateAttributes=''  IntegratorStateMustResolveToSignalObject=off  IntegratorRTWStateStorageClass=Auto  FilterContinuousStateAttributes=''  FilterStateMustResolveToSignalObject=off  FilterRTWStateStorageClass=Auto  ParallelPVariant=InternalParameters  IdealPVariant=Disabled  IVariant=InternalParameters  DVariant=Disabled  IntegratorVariant=Continuous  SatVariant=Disabled  AWVariant=Passthrough  PCopyVariant=Disabled  TRVariant=Disabled  FdbkBlocksVariant=Forward  IdealPFdbkVariant=Disabled  SatFdbkVariant=Disabled  DerivativeFilterVariant=Disabled  NVariant=Disabled  NCopyVariant=Disabled_SignalSpec  FilterICVariant=Disabled  IntegratorICVariant=InternalICs  ExternalResetVariant=Disabled  TRSumVariant=Passthrough  SumFdbkVariant=Disabled  SumVariant=Sum_PI  TsampFilterVariant=InternalTs  TsampNgainVariant=Passthrough  TsampIntegralVariant=Passthrough
  Saturation : Saturate  UpperLimit=Ubat  LowerLimit=0
  Sum : Sum  Inputs=++|
  Sum1 : Sum  Inputs=|-+
  Uch_ref : Outport  InitialOutput=0
  wires:
  PID Controller/1 -> Sum/2
  Uc/1 -> Sum/1
  Sum1/1 -> PID Controller/1
  IL_ref/1 -> Sum1/2
  IL/1 -> Sum1/1
  Sum/1 -> Saturation/1
  Saturation/1 -> Uch_ref/1

== system Buck_DCM_s/Load ==
  w : Inport
  Load : Step  After=30  SampleTime=0
  Terminator : Terminator
  Mc : Outport  InitialOutput=0  VectorParamsAs1DForOutWhenUnconnected=off
  wires:
  w/1 -> Terminator/1
  Load/1 -> Mc/1

== system Buck_DCM_s/Load3 ==
  Uc : Inport
  Gain : Gain  Commented=on  Gain=1/10
  Product : Product
  Step : Step  Time=10  After=10  SampleTime=0
  iload : Outport  InitialOutput=0  VectorParamsAs1DForOutWhenUnconnected=off
  wires:
  Uc/1 -> Product/1
  Product/1 -> iload/1
  Step/1 -> Product/2

== system Buck_DCM_s/Load4 ==
  Wdcm : Inport
  Terminator : Terminator
  w_ref1 : Step  Time=5  After=30  SampleTime=0
  Tload : Outport  InitialOutput=0  VectorParamsAs1DForOutWhenUnconnected=off
  wires:
  Wdcm/1 -> Terminator/1
  w_ref1/1 -> Tload/1

== system Buck_DCM_s/Mc Estimation ==
  Iu : Inport
  w : Inport  Port=2
  Gain1 : Gain  Gain=Kphi
  Sum : Sum  Inputs=|+-
  Transfer Fcn : TransferFcn  Numerator=[J 0]  Denominator=[0.001 1]
  Mc : Outport  InitialOutput=0  VectorParamsAs1DForOutWhenUnconnected=off
  wires:
  Transfer Fcn/1 -> Sum/2
  w/1 -> Transfer Fcn/1
  Iu/1 -> Gain1/1
  Gain1/1 -> Sum/1
  Sum/1 -> Mc/1

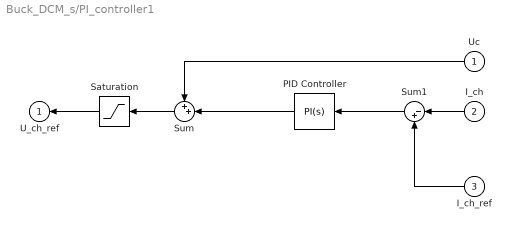
== system Buck_DCM_s/PI_controller1 ==
  Uc : Inport
  I_ch : Inport  Port=2
  "I_ch_ref " : Inport  Port=3
  PID Controller : simulink/Continuous/PID Controller  Controller=PI  Form=Parallel  TimeDomain=Continuous-time  UseExternalTs=off  SampleTime=-1  IntegratorMethod=Forward Euler  FilterMethod=Forward Euler  ControllerParametersSource=internal  P=Kp_IL  I=Ki_IL  D=0  UseFilter=on  N=100  TunerSelectOption=Transfer Function Based (PID Tuner App)  InitialConditionSource=internal  InitialConditionForIntegrator=0  InitialConditionForFilter=0  DifferentiatorICPrevScaledInput=0  ExternalReset=none  TrackingMode=off  Kt=1  LimitOutput=off  UpperSaturationLimit=inf  LowerSaturationLimit=-inf  LinearizeAsGain=on  AntiWindupMode=none  Kb=1  POutMin=[]  POutMax=[]  IOutMin=[]  IOutMax=[]  DOutMin=[]  DOutMax=[]  NOutMin=[]  NOutMax=[]  SumOutMin=[]  SumOutMax=[]  SaturationOutMin=[]  SaturationOutMax=[]  PParamMin=[]  PParamMax=[]  IParamMin=[]  IParamMax=[]  DParamMin=[]  DParamMax=[]  NParamMin=[]  NParamMax=[]  KbParamMin=[]  KbParamMax=[]  KtParamMin=[]  KtParamMax=[]  KbOutMin=[]  KbOutMax=[]  KtOutMin=[]  KtOutMax=[]  IntegratorOutMin=[]  IntegratorOutMax=[]  FilterOutMin=[]  FilterOutMax=[]  SumI1OutMin=[]  SumI1OutMax=[]  SumI2OutMin=[]  SumI2OutMax=[]  SumI3OutMin=[]  SumI3OutMax=[]  SumI4OutMin=[]  SumI4OutMax=[]  SumDOutMin=[]  SumDOutMax=[]  DifferentiatorOutMin=[]  DifferentiatorOutMax=[]  FilterDiffOutCoefMin=[]  FilterDiffOutCoefMax=[]  ReciprocalOutMin=[]  ReciprocalOutMax=[]  SumDenOutMin=[]  SumDenOutMax=[]  SumNumOutMin=[]  SumNumOutMax=[]  DivideOutMin=[]  DivideOutMax=[]  UdiffTsProdOutMin=[]  UdiffTsProdOutMax=[]  NTsProdOutMin=[]  NTsProdOutMax=[]  UintegralTsProdOutMin=[]  UintegralTsProdOutMax=[]  UngainTsProdOutMin=[]  UngainTsProdOutMax=[]  IntegratorContinuousStateAttributes=''  IntegratorStateMustResolveToSignalObject=off  IntegratorRTWStateStorageClass=Auto  FilterContinuousStateAttributes=''  FilterStateMustResolveToSignalObject=off  FilterRTWStateStorageClass=Auto  ParallelPVariant=InternalParameters  IdealPVariant=Disabled  IVariant=InternalParameters  DVariant=Disabled  IntegratorVariant=Continuous  SatVariant=Disabled  AWVariant=Passthrough  PCopyVariant=Disabled  TRVariant=Disabled  FdbkBlocksVariant=Forward  IdealPFdbkVariant=Disabled  SatFdbkVariant=Disabled  DerivativeFilterVariant=Disabled  NVariant=Disabled  NCopyVariant=Disabled_SignalSpec  FilterICVariant=Disabled  IntegratorICVariant=InternalICs  ExternalResetVariant=Disabled  TRSumVariant=Passthrough  SumFdbkVariant=Disabled  SumVariant=Sum_PI  TsampFilterVariant=InternalTs  TsampNgainVariant=Passthrough  TsampIntegralVariant=Passthrough
  Saturation : Saturate  UpperLimit=Ubat  LowerLimit=0
  Sum : Sum  Inputs=++|
  Sum1 : Sum  Inputs=|-+
  U_ch_ref : Outport  InitialOutput=0
  wires:
  PID Controller/1 -> Sum/2
  Sum/1 -> Saturation/1
  Uc/1 -> Sum/1
  Sum1/1 -> PID Controller/1
  "I_ch_ref "/1 -> Sum1/2
  I_ch/1 -> Sum1/1
  Saturation/1 -> U_ch_ref/1

== system Buck_DCM_s/PWM ==
  Ubat : Inport
  Uch_ref : Inport  Port=2
  Divide : Product  Inputs=/*
  PWM Generator (DC-DC) : powerlib_meascontrol/Pulse & Signal Generators/PWM Generator (DC-DC)  Commented=through  Fsw=10000  Ts=0
  PWM : Outport
  wires:
  PWM Generator (DC-DC)/1 -> PWM/1
  Ubat/1 -> Divide/1
  Uch_ref/1 -> Divide/2
  Divide/1 -> PWM Generator (DC-DC)/1

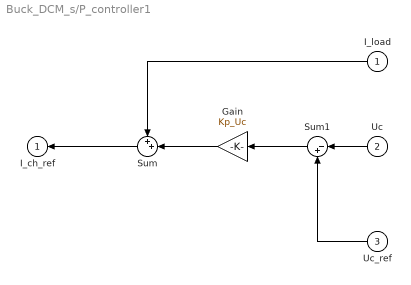
== system Buck_DCM_s/P_controller1 ==
  I_load : Inport
  Uc : Inport  Port=2
  Uc_ref : Inport  Port=3
  Gain : Gain  Gain=Kp_Uc
  Sum : Sum  Inputs=++|
  Sum1 : Sum  Inputs=|-+
  I_ch_ref : Outport  InitialOutput=0
  wires:
  Uc/1 -> Sum1/1
  Uc_ref/1 -> Sum1/2
  Sum1/1 -> Gain/1
  Gain/1 -> Sum/2
  I_load/1 -> Sum/1
  Sum/1 -> I_ch_ref/1

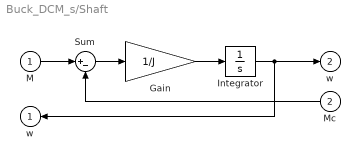
== system Buck_DCM_s/Shaft ==
  M : Inport
  Mc : Inport  Port=2
  Gain : Gain  Gain=1/J
  Integrator : Integrator  InitialCondition=0.001
  Sum : Sum  Inputs=|+-
  w : Outport  InitialOutput=0  VectorParamsAs1DForOutWhenUnconnected=off
  "w " : Outport  Port=2  InitialOutput=0  VectorParamsAs1DForOutWhenUnconnected=off
  wires:
  M/1 -> Sum/1
  Mc/1 -> Sum/2
  Sum/1 -> Gain/1
  Integrator/1 -> "w "/1, w/1
  Gain/1 -> Integrator/1

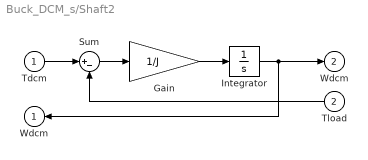
== system Buck_DCM_s/Shaft2 ==
  Tdcm : Inport
  Tload : Inport  Port=2
  Gain : Gain  Gain=1/J
  Integrator : Integrator  InitialCondition=0.001
  Sum : Sum  Inputs=|+-
  Wdcm : Outport  InitialOutput=0  VectorParamsAs1DForOutWhenUnconnected=off
  "Wdcm " : Outport  Port=2  InitialOutput=0  VectorParamsAs1DForOutWhenUnconnected=off
  wires:
  Tdcm/1 -> Sum/1
  Tload/1 -> Sum/2
  Sum/1 -> Gain/1
  Integrator/1 -> "Wdcm "/1, Wdcm/1
  Gain/1 -> Integrator/1

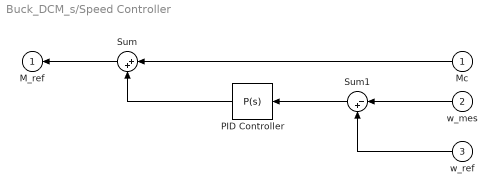
== system Buck_DCM_s/Speed Controller ==
  Mc : Inport
  w_mes : Inport  Port=2
  w_ref : Inport  Port=3
  PID Controller : simulink/Continuous/PID Controller  Controller=P  Form=Parallel  TimeDomain=Continuous-time  UseExternalTs=off  SampleTime=-1  IntegratorMethod=Forward Euler  FilterMethod=Forward Euler  ControllerParametersSource=internal  P=Kp_W  I=Ki_W  D=0  UseFilter=on  N=100  TunerSelectOption=Transfer Function Based (PID Tuner App)  InitialConditionSource=internal  InitialConditionForIntegrator=0  InitialConditionForFilter=0  DifferentiatorICPrevScaledInput=0  ExternalReset=none  TrackingMode=off  Kt=1  LimitOutput=off  UpperSaturationLimit=inf  LowerSaturationLimit=-inf  LinearizeAsGain=on  AntiWindupMode=none  Kb=1  POutMin=[]  POutMax=[]  IOutMin=[]  IOutMax=[]  DOutMin=[]  DOutMax=[]  NOutMin=[]  NOutMax=[]  SumOutMin=[]  SumOutMax=[]  SaturationOutMin=[]  SaturationOutMax=[]  PParamMin=[]  PParamMax=[]  IParamMin=[]  IParamMax=[]  DParamMin=[]  DParamMax=[]  NParamMin=[]  NParamMax=[]  KbParamMin=[]  KbParamMax=[]  KtParamMin=[]  KtParamMax=[]  KbOutMin=[]  KbOutMax=[]  KtOutMin=[]  KtOutMax=[]  IntegratorOutMin=[]  IntegratorOutMax=[]  FilterOutMin=[]  FilterOutMax=[]  SumI1OutMin=[]  SumI1OutMax=[]  SumI2OutMin=[]  SumI2OutMax=[]  SumI3OutMin=[]  SumI3OutMax=[]  SumI4OutMin=[]  SumI4OutMax=[]  SumDOutMin=[]  SumDOutMax=[]  DifferentiatorOutMin=[]  DifferentiatorOutMax=[]  FilterDiffOutCoefMin=[]  FilterDiffOutCoefMax=[]  ReciprocalOutMin=[]  ReciprocalOutMax=[]  SumDenOutMin=[]  SumDenOutMax=[]  SumNumOutMin=[]  SumNumOutMax=[]  DivideOutMin=[]  DivideOutMax=[]  UdiffTsProdOutMin=[]  UdiffTsProdOutMax=[]  NTsProdOutMin=[]  NTsProdOutMax=[]  UintegralTsProdOutMin=[]  UintegralTsProdOutMax=[]  UngainTsProdOutMin=[]  UngainTsProdOutMax=[]  IntegratorContinuousStateAttributes=''  IntegratorStateMustResolveToSignalObject=off  IntegratorRTWStateStorageClass=Auto  FilterContinuousStateAttributes=''  FilterStateMustResolveToSignalObject=off  FilterRTWStateStorageClass=Auto  ParallelPVariant=InternalParameters  IdealPVariant=Disabled  IVariant=Disabled  DVariant=Disabled  IntegratorVariant=Disabled  SatVariant=Disabled  AWVariant=Disabled  PCopyVariant=Disabled  TRVariant=Disabled  FdbkBlocksVariant=Forward  IdealPFdbkVariant=Disabled  SatFdbkVariant=Disabled  DerivativeFilterVariant=Disabled  NVariant=Disabled  NCopyVariant=Disabled_SignalSpec  FilterICVariant=Disabled  IntegratorICVariant=Disabled  ExternalResetVariant=Disabled  TRSumVariant=Passthrough  SumFdbkVariant=Disabled  SumVariant=Passthrough_P  TsampFilterVariant=InternalTs  TsampNgainVariant=Passthrough  TsampIntegralVariant=Disabled_SignalSpec
  Sum : Sum  Inputs=|++
  Sum1 : Sum  Inputs=|-+
  M_ref : Outport  InitialOutput=0  VectorParamsAs1DForOutWhenUnconnected=off
  wires:
  Sum/1 -> M_ref/1
  w_mes/1 -> Sum1/1
  w_ref/1 -> Sum1/2
  Sum1/1 -> PID Controller/1
  PID Controller/1 -> Sum/2
  Mc/1 -> Sum/1

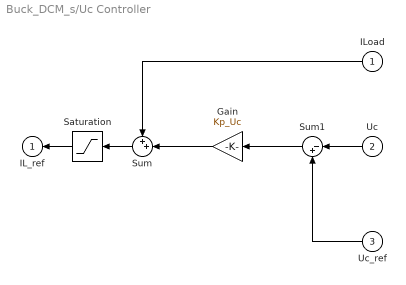
== system Buck_DCM_s/Uc Controller ==
  ILoad : Inport
  Uc : Inport  Port=2
  Uc_ref : Inport  Port=3
  Gain : Gain  Gain=Kp_Uc
  Saturation : Saturate  UpperLimit=10000  LowerLimit=0
  Sum : Sum  Inputs=++|
  Sum1 : Sum  Inputs=|-+
  IL_ref : Outport  InitialOutput=0
  wires:
  Uc/1 -> Sum1/1
  Uc_ref/1 -> Sum1/2
  Sum1/1 -> Gain/1
  Gain/1 -> Sum/2
  ILoad/1 -> Sum/1
  Sum/1 -> Saturation/1
  Saturation/1 -> IL_ref/1

== system Buck_DCM_s/Uch->m1 ==
  Ud0_mes : Inport
  Uch_ref : Inport  Port=2
  Divide : Product  Inputs=/*
  Saturation : Saturate  UpperLimit=1  LowerLimit=-1
  m : Outport  InitialOutput=0  VectorParamsAs1DForOutWhenUnconnected=off
  wires:
  Divide/1 -> Saturation/1
  Ud0_mes/1 -> Divide/1
  Uch_ref/1 -> Divide/2
  Saturation/1 -> m/1

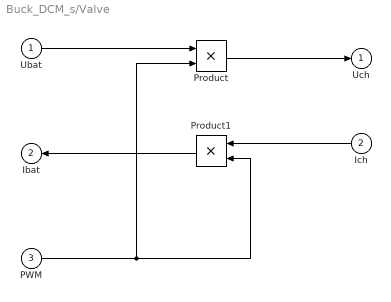
== system Buck_DCM_s/Valve ==
  Ubat : Inport
  Ich : Inport  Port=2
  PWM : Inport  Port=3
  Product : Product
  Product1 : Product
  Uch : Outport  InitialOutput=0  VectorParamsAs1DForOutWhenUnconnected=off
  Ibat : Outport  Port=2  InitialOutput=0  VectorParamsAs1DForOutWhenUnconnected=off
  wires:
  Product/1 -> Uch/1
  Ubat/1 -> Product/1
  PWM/1 -> Product1/2, Product/2
  Ich/1 -> Product1/1
  Product1/1 -> Ibat/1

== system Buck_DCM_s/Valve2 ==
  Ubat : Inport
  Ich : Inport  Port=2
  PWM : Inport  Port=3
  Product : Product
  Product1 : Product
  Uch : Outport  InitialOutput=0  VectorParamsAs1DForOutWhenUnconnected=off
  Ibat : Outport  Port=2  InitialOutput=0  VectorParamsAs1DForOutWhenUnconnected=off
  wires:
  Product/1 -> Uch/1
  Ubat/1 -> Product/1
  PWM/1 -> Product1/2, Product/2
  Ich/1 -> Product1/1
  Product1/1 -> Ibat/1

== system Buck_DCM_s/Winding ==
  Uch : Inport
  Uc : Inport  Port=2
  Add : Sum  Inputs=+-
  Transfer Fcn : TransferFcn  Denominator=[L rL]
  IL : Outport  InitialOutput=0  VectorParamsAs1DForOutWhenUnconnected=off
  "IL " : Outport  Port=2  InitialOutput=0  VectorParamsAs1DForOutWhenUnconnected=off
  wires:
  Uch/1 -> Add/1
  Transfer Fcn/1 -> "IL "/1, IL/1
  Add/1 -> Transfer Fcn/1
  Uc/1 -> Add/2

== system Buck_DCM_s/Winding2 ==
  Uch : Inport
  Uc : Inport  Port=2
  Sum : Sum  Inputs=|+-
  Transfer Fcn : TransferFcn  Denominator=[L rL]
  Ich : Outport  InitialOutput=0  VectorParamsAs1DForOutWhenUnconnected=off
  Ich1 : Outport  Port=2  InitialOutput=0  VectorParamsAs1DForOutWhenUnconnected=off
  wires:
  Uch/1 -> Sum/1
  Transfer Fcn/1 -> Ich1/1, Ich/1
  Sum/1 -> Transfer Fcn/1
  Uc/1 -> Sum/2

== system Buck_DCM_s/chopper ==
  "Ubat " : Inport
  idcm : Inport  Port=2
  m : Inport  Port=3
  Divide : Product  Inputs=**
  Divide1 : Product  Inputs=**
  Uch : Outport  InitialOutput=0  VectorParamsAs1DForOutWhenUnconnected=off
  ibat : Outport  Port=2  InitialOutput=0  VectorParamsAs1DForOutWhenUnconnected=off
  wires:
  m/1 -> Divide/2, Divide1/1
  Divide1/1 -> Uch/1
  "Ubat "/1 -> Divide1/2
  Divide/1 -> ibat/1
  idcm/1 -> Divide/1

== system Buck_DCM_s/converter EM2 ==
  Tm_ref : Inport
  Gain : Gain  Gain=1/Kphi
  Saturation : Saturate  UpperLimit=5*Idm  LowerLimit=-5*Idm
  Idcm_ref : Outport  InitialOutput=0  VectorParamsAs1DForOutWhenUnconnected=off
  wires:
  Tm_ref/1 -> Gain/1
  Gain/1 -> Saturation/1
  Saturation/1 -> Idcm_ref/1

== system Buck_DCM_s/converter inversion2 ==
  U_bat : Inport
  U_ch_ref : Inport  Port=2
  Divide : Product  Inputs=/*
  PWM Generator (DC-DC) : powerlib_meascontrol/Pulse & Signal Generators/PWM Generator (DC-DC)  Commented=through  Fsw=5000  Ts=0
  PWM : Outport
  wires:
  U_bat/1 -> Divide/1
  U_ch_ref/1 -> Divide/2
  PWM Generator (DC-DC)/1 -> PWM/1
  Divide/1 -> PWM Generator (DC-DC)/1

== system Buck_DCM_s/current controller 2 ==
  Idcm_mes : Inport
  Edcm_mes : Inport  Port=2
  Idcm_ref : Inport  Port=3
  PID Controller : simulink/Continuous/PID Controller  Controller=PI  Form=Parallel  TimeDomain=Continuous-time  UseExternalTs=off  SampleTime=-1  IntegratorMethod=Forward Euler  FilterMethod=Forward Euler  ControllerParametersSource=internal  P=Kp_I  I=Ki_I  D=0  UseFilter=on  N=100  TunerSelectOption=Transfer Function Based (PID Tuner App)  InitialConditionSource=internal  InitialConditionForIntegrator=0  InitialConditionForFilter=0  DifferentiatorICPrevScaledInput=0  ExternalReset=none  IgnoreLimit=on  TrackingMode=off  Kt=1  LimitOutput=off  UpperSaturationLimit=inf  LowerSaturationLimit=-inf  LinearizeAsGain=on  AntiWindupMode=none  Kb=1  POutMin=[]  POutMax=[]  IOutMin=[]  IOutMax=[]  DOutMin=[]  DOutMax=[]  NOutMin=[]  NOutMax=[]  SumOutMin=[]  SumOutMax=[]  SaturationOutMin=[]  SaturationOutMax=[]  PParamMin=[]  PParamMax=[]  IParamMin=[]  IParamMax=[]  DParamMin=[]  DParamMax=[]  NParamMin=[]  NParamMax=[]  KbParamMin=[]  KbParamMax=[]  KtParamMin=[]  KtParamMax=[]  KbOutMin=[]  KbOutMax=[]  KtOutMin=[]  KtOutMax=[]  IntegratorOutMin=[]  IntegratorOutMax=[]  FilterOutMin=[]  FilterOutMax=[]  SumI1OutMin=[]  SumI1OutMax=[]  SumI2OutMin=[]  SumI2OutMax=[]  SumI3OutMin=[]  SumI3OutMax=[]  SumI4OutMin=[]  SumI4OutMax=[]  SumDOutMin=[]  SumDOutMax=[]  DifferentiatorOutMin=[]  DifferentiatorOutMax=[]  FilterDiffOutCoefMin=[]  FilterDiffOutCoefMax=[]  ReciprocalOutMin=[]  ReciprocalOutMax=[]  SumDenOutMin=[]  SumDenOutMax=[]  SumNumOutMin=[]  SumNumOutMax=[]  DivideOutMin=[]  DivideOutMax=[]  UdiffTsProdOutMin=[]  UdiffTsProdOutMax=[]  NTsProdOutMin=[]  NTsProdOutMax=[]  UintegralTsProdOutMin=[]  UintegralTsProdOutMax=[]  UngainTsProdOutMin=[]  UngainTsProdOutMax=[]  IntegratorContinuousStateAttributes=''  IntegratorStateMustResolveToSignalObject=off  IntegratorRTWStateStorageClass=Auto  FilterContinuousStateAttributes=''  FilterStateMustResolveToSignalObject=off  FilterRTWStateStorageClass=Auto  ParallelPVariant=InternalParameters  IdealPVariant=Disabled  IVariant=InternalParameters  DVariant=Disabled  IntegratorVariant=Continuous  SatVariant=Disabled  AWVariant=Passthrough  PCopyVariant=Disabled  TRVariant=Disabled  FdbkBlocksVariant=Forward  IdealPFdbkVariant=Disabled  SatFdbkVariant=Disabled  DerivativeFilterVariant=Disabled  NVariant=Disabled  NCopyVariant=Disabled_SignalSpec  FilterICVariant=Disabled  IntegratorICVariant=InternalICs  ExternalResetVariant=Disabled  TRSumVariant=Passthrough  SumFdbkVariant=Disabled  SumVariant=Sum_PI  TsampFilterVariant=InternalTs  TsampNgainVariant=Passthrough  TsampIntegralVariant=Passthrough
  Sum : Sum  Inputs=|++
  Sum1 : Sum  Inputs=|-+
  Uch_ref : Outport  InitialOutput=0  VectorParamsAs1DForOutWhenUnconnected=off
  wires:
  Edcm_mes/1 -> Sum/1
  Sum/1 -> Uch_ref/1
  Idcm_mes/1 -> Sum1/1
  Sum1/1 -> PID Controller/1
  PID Controller/1 -> Sum/2
  Idcm_ref/1 -> Sum1/2

== system Buck_DCM_s/speed controller2 ==
  Tload : Inport
  wm_mes : Inport  Port=2
  wm_ref : Inport  Port=3
  PID Controller : simulink/Continuous/PID Controller  Controller=P  Form=Parallel  TimeDomain=Continuous-time  UseExternalTs=off  SampleTime=-1  IntegratorMethod=Forward Euler  FilterMethod=Forward Euler  ControllerParametersSource=internal  P=Kp_W  I=Ki_W  D=0  UseFilter=on  N=100  TunerSelectOption=Transfer Function Based (PID Tuner App)  InitialConditionSource=internal  InitialConditionForIntegrator=0  InitialConditionForFilter=0  DifferentiatorICPrevScaledInput=0  ExternalReset=none  TrackingMode=off  Kt=1  LimitOutput=off  UpperSaturationLimit=inf  LowerSaturationLimit=-inf  LinearizeAsGain=on  AntiWindupMode=none  Kb=1  POutMin=[]  POutMax=[]  IOutMin=[]  IOutMax=[]  DOutMin=[]  DOutMax=[]  NOutMin=[]  NOutMax=[]  SumOutMin=[]  SumOutMax=[]  SaturationOutMin=[]  SaturationOutMax=[]  PParamMin=[]  PParamMax=[]  IParamMin=[]  IParamMax=[]  DParamMin=[]  DParamMax=[]  NParamMin=[]  NParamMax=[]  KbParamMin=[]  KbParamMax=[]  KtParamMin=[]  KtParamMax=[]  KbOutMin=[]  KbOutMax=[]  KtOutMin=[]  KtOutMax=[]  IntegratorOutMin=[]  IntegratorOutMax=[]  FilterOutMin=[]  FilterOutMax=[]  SumI1OutMin=[]  SumI1OutMax=[]  SumI2OutMin=[]  SumI2OutMax=[]  SumI3OutMin=[]  SumI3OutMax=[]  SumI4OutMin=[]  SumI4OutMax=[]  SumDOutMin=[]  SumDOutMax=[]  DifferentiatorOutMin=[]  DifferentiatorOutMax=[]  FilterDiffOutCoefMin=[]  FilterDiffOutCoefMax=[]  ReciprocalOutMin=[]  ReciprocalOutMax=[]  SumDenOutMin=[]  SumDenOutMax=[]  SumNumOutMin=[]  SumNumOutMax=[]  DivideOutMin=[]  DivideOutMax=[]  UdiffTsProdOutMin=[]  UdiffTsProdOutMax=[]  NTsProdOutMin=[]  NTsProdOutMax=[]  UintegralTsProdOutMin=[]  UintegralTsProdOutMax=[]  UngainTsProdOutMin=[]  UngainTsProdOutMax=[]  IntegratorContinuousStateAttributes=''  IntegratorStateMustResolveToSignalObject=off  IntegratorRTWStateStorageClass=Auto  FilterContinuousStateAttributes=''  FilterStateMustResolveToSignalObject=off  FilterRTWStateStorageClass=Auto  ParallelPVariant=InternalParameters  IdealPVariant=Disabled  IVariant=Disabled  DVariant=Disabled  IntegratorVariant=Disabled  SatVariant=Disabled  AWVariant=Disabled  PCopyVariant=Disabled  TRVariant=Disabled  FdbkBlocksVariant=Forward  IdealPFdbkVariant=Disabled  SatFdbkVariant=Disabled  DerivativeFilterVariant=Disabled  NVariant=Disabled  NCopyVariant=Disabled_SignalSpec  FilterICVariant=Disabled  IntegratorICVariant=Disabled  ExternalResetVariant=Disabled  TRSumVariant=Passthrough  SumFdbkVariant=Disabled  SumVariant=Passthrough_P  TsampFilterVariant=InternalTs  TsampNgainVariant=Passthrough  TsampIntegralVariant=Disabled_SignalSpec
  Sum : Sum  Inputs=|++
  Sum1 : Sum  Inputs=|-+
  Tm_ref : Outport  InitialOutput=0  VectorParamsAs1DForOutWhenUnconnected=off
  wires:
  Sum/1 -> Tm_ref/1
  wm_mes/1 -> Sum1/1
  wm_ref/1 -> Sum1/2
  Sum1/1 -> PID Controller/1
  PID Controller/1 -> Sum/2
  Tload/1 -> Sum/1

== system Buck_DCM_s/winding ==
  Uch : Inport
  Edcm : Inport  Port=2
  1/(Ls+R) : TransferFcn  Denominator=[Lu Ru]
  Sum : Sum  Inputs=|+-
  "idcm " : Outport  InitialOutput=0  VectorParamsAs1DForOutWhenUnconnected=off
  idcm : Outport  Port=2  InitialOutput=0  VectorParamsAs1DForOutWhenUnconnected=off
  wires:
  Uch/1 -> Sum/1
  Edcm/1 -> Sum/2
  Sum/1 -> 1/(Ls+R)/1
  1/(Ls+R)/1 -> idcm/1, "idcm "/1
